simulink model "Start_Stop_ECU"  (R2023b)
settings: Solver=FixedStepDiscrete  StartTime=0.0  StopTime=24  FixedStep=0.01  RelTol=1e-3
model workspace (MATLAB code in the model file):
  | % Girişler (Inputs)
  | Start_Permission = 0;
  | Start_Button = 0;
  | Motor_RPM = 0;
  | 
  | % Çıkışlar (Outputs)
  | Mars_Motoru = 0;
  | Ignition_State = 0;
  | Target_RPM = 0;
settings Model: PacingRate=0.320000  Creator=BERKE  LastModifiedBy=BERKE
settings ConfigComp: CovEnable=on  RecordCoverage=on  CovModelRefEnable=on

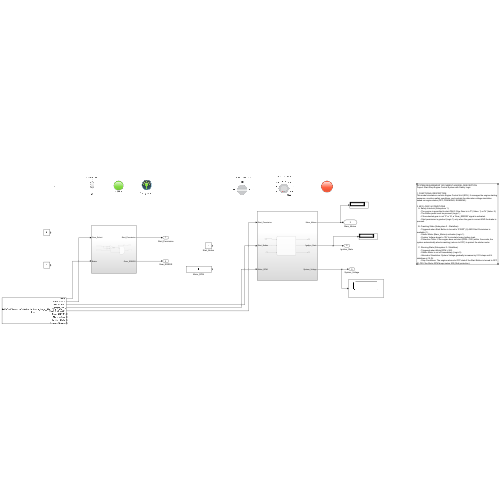
[thumbnail: Simulink's stored preview of the top-level diagram]
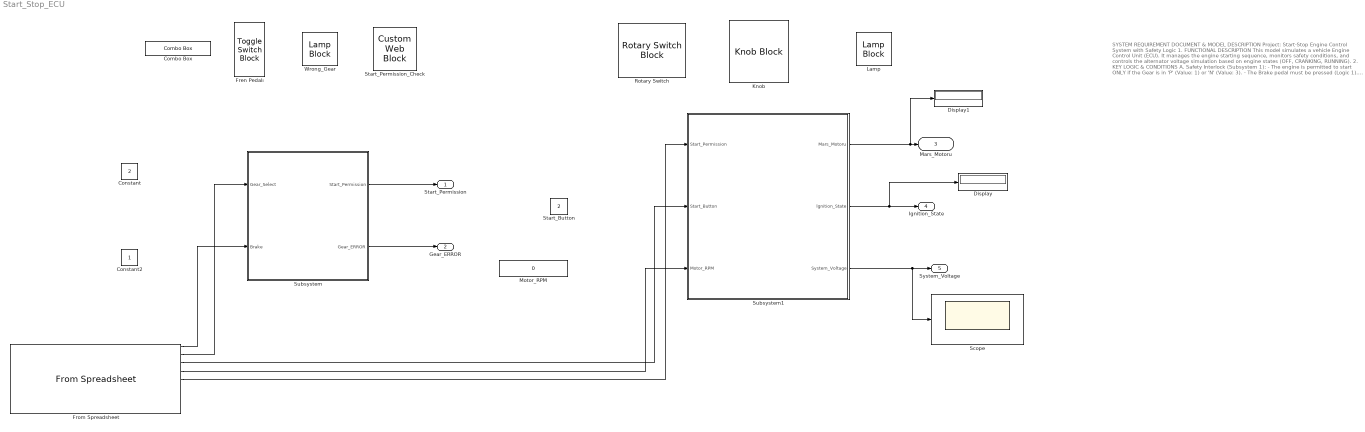
== system Start_Stop_ECU ==
  note: SYSTEM REQUIREMENT DOCUMENT & MODEL DESCRIPTION
      | Project: Start-Stop Engine Control System with Safety Logic
      |
      | 1. FUNCTIONAL DESCRIPTION
      | This model simulates a vehicle Engine Control Unit (ECU). It manages the engine starting sequence, monitors safety conditions, and controls the alternator voltage simulation based on engine states (OFF, CRANKING, RUNNING).
      |
      | 2. KEY LOGIC & CONDITIONS
      |    A. Safety Interlock (Subsystem 1):
      |       - The engine is permitted to start ONLY if the Gear is in 'P' (Value: 1) or 'N' (Value: 3).
      |       - The Brake pedal must be pressed (Logic 1).
      |       - If the selected gear is not 'P' or 'N', a 'Gear_ERROR' signal is activated.
      |       - Start permission is granted (Logic 1) only when the gear is correct AND the brake is pressed.
      |
      |    B. Cranking State (Subsystem 2 - Stateflow):
      |       - Triggered when Start Button is turned to 'START' (2) AND Start Permission is available (1).
      |       - Starter Motor (Mars_Motoru) activates (Logic 1).
      |       - System Voltage drops to 10V to simulate heavy battery load.
      |       - Protection Timer: If the engine does not start (RPM < 500) within 3 seconds, the system automatically aborts cranking (returns to OFF) to protect the starter motor.
      |
      |    C. Running State (Subsystem 2 - Stateflow):
      |       - Triggered when Motor RPM > 500.
      |       - Starter Motor is cut off immediately (Logic 0).
      |       - Alternator Simulation: System Voltage gradually increases by 0.5V steps until it stabilizes at 12.5V.
      |       - Stop Conditions: The engine returns to OFF state if the Start Button is turned to OFF (0) OR if the Motor RPM drops below 500 (Stall protection).
  Combo Box : ComboBox  LabelPosition=Hide  SelectedLabel=R
      settings: Values={{'P', 'R', 'N', 'D'}, [1 2 3 4]}
  Constant : Constant  Value=2
  Constant2 : Constant
  Display : Display
  Display1 : Display
  Fren Pedalı : ToggleSwitchBlock
      settings: Values={{'Off', 'On'}, [0 1]}
  From Spreadsheet : FromSpreadsheet  FileName=C:\Users\BERKE\OneDrive\Masaüstü\simulink\Berke_Girgin_290206067_HW2_Coverage.xlsx
  Knob : KnobBlock  ScaleMax=5000
  Lamp : LampBlock  LabelPosition=Hide
  "Motor_RPM " : Constant  Value=0
  Rotary Switch : RotarySwitchBlock
      settings: Values={{'Off', 'IGN', 'START'}, [0 1 2]}
  Scope : Scope
  Start_Button : Constant  Value=2  SampleTime=-1
  Start_Permission_Check : CustomWebBlock  LabelPosition=Bottom  ShowInitialText=on  Configuration="{\"components\":[{\"name\":\"BackgroundImageComponent\",\"settings\":{\"image\":{\"size\":[150,150],\"src\":\"data:image\\/svg+xml;base64,PHN2ZyB4bWxucz0iaHR0cDovL3d3dy53My5vcmcvMjAwMC9zdmciIHhtbG5zOnhsaW5rPSJodHRwOi8vd3d3LnczLm9yZy8xOTk5L3hsaW5rIiB2aWV3Qm94PSIwIDAgNTAwIDUwMCI+PGRlZnM+PHN0eWxlPi5he2ZpbGw6dXJsKCNhKTt9LmJ7ZmlsbDp1cmwoI2IpO30uY3tmaWxsOnVybCgjYyk7fTwvc3R5bGU+PHJhZGlhbEdyYWRpZW50IGlkPSJhIiBjeD0iMjgzLjg0IiBjeT0iLTQ2Ni4zNyIgcj0iMzc1Ljc1IiBncmFkaWVudFRyYW5zZm9ybT0ibWF0cml4KDEuMzksIDAsIDAsIC0xLjM5LCAtMTUzLjU2LCAtNjQ0LjA4KSIg ...(+2088 chars)\",\"srcOrientation\":\"Right\"},\"position\":[0,0,1,1],\"scaleMode\":\"0\"}},{\"name\":\"LampStateComponent\",\"settings\":{\"position\":[0,0,1,1],\"states\":[{\"icon\":{\"customSrc\":\"data:image\\/svg+xml;base64,PHN2ZyBpZD0iTGF5ZXJfMSIgZGF0YS1uYW1lPSJMYXllciAxIiB4bWxucz0iaHR0cDovL3d3dy53My5vcmcvMjAwMC9zdmciIHZpZXdCb3g9IjAgMCA0MTEgNDU4Ij48ZGVmcz48c3R5bGU+LmNscy0xe2ZpbGw6I2ZkZjhjMTt9LmNscy0ye2ZpbGw6I2ZlZTEwMDt9LmNscy0ze2ZpbGw6IzIzMWYyMDt9LmNscy00e2ZpbGw6I2EwOWY5Zjt9LmNscy00LC5jbHMtNSwuY2xzLTZ7c3Ryb2tlOiMyMzFmMjA7c3Ryb2tlLW1pdGVybGltaXQ6MTA7fS5jbHMtNXtmaWxsOiNmZmY7fS5jbHMtNntmaWxsOm5vbmU7fTwvc3R5bGU+PC9kZWZz ...(+5168 chars)\",\"id\":-1,\"srcOrientation\":\"Right\",\"type\":\"custom\"},\"iconScale\":0.8,\"metadata\":{},\"overlayType\":\"intersect\",\"shape\":{\"color\":[0.725,0,0],\"opacity\":1,\"position\":[0.1,0.1,0.8,0.8],\"type\":\"ellipse\"},\"value\":[]},{\"icon\":{\"customSrc\":\"data:image\\/svg+xml;base64,PHN2ZyBpZD0iTGF5ZXJfMSIgZGF0YS1uYW1lPSJMYXllciAxIiB4bWxucz0iaHR0cDovL3d3dy53My5vcmcvMjAwMC9zdmciIHZpZXdCb3g9IjAgMCA0MTEgNDU4Ij48ZGVmcz48c3R5bGU+LmNscy0xe2ZpbGw6I2ZkZjhjMTt9LmNscy0ye2ZpbGw6I2ZlZTEwMDt9LmNscy0ze2ZpbGw6IzIzMWYyMDt9LmNscy00e2ZpbGw6I2EwOWY5Zjt9LmNscy00LC5jbHMtNSwuY2xzLTZ7c3Ryb2tlOiMyMzFmMjA7c3Ryb2tlLW1pdGVybGltaXQ6MTA7fS5jbHMtNXtmaWxsOiNmZmY7fS5jbHMtNntmaWxsOm5vbmU7fTwvc3R5bGU+PC9kZWZz ...(+5168 chars)\",\"id\":-1,\"srcOrientation\":\"Right\",\"type\":\"custom\"},\"iconScale\":0.8,\"metadata\":{\"useDefaults\":{\"customIcon\":true,\"icon\":true,\"overlayType\":true,\"shape\":true,\"sizeAndPosition\":true}},\"overlayType\":\"intersect\",\"shape\":{\"color\":[0.6352941176470588,0.0784313725490196,0.1843137254901961],\"opacity\":1,\"position\":[0.1,0.1,0.8,0.8],\"type\":\"ellipse\"},\"value\":\"0\"},{\"icon\":{\"customSrc\":\"data:image\\/svg+xml;base64,PHN2ZyBpZD0iTGF5ZXJfMSIgZGF0YS1uYW1lPSJMYXllciAxIiB4bWxucz0iaHR0cDovL3d3dy53My5vcmcvMjAwMC9zdmciIHZpZXdCb3g9IjAgMCA0MTEgNDU4Ij48ZGVmcz48c3R5bGU+LmNscy0xe2ZpbGw6I2ZkZjhjMTt9LmNscy0ye2ZpbGw6I2ZlZTEwMDt9LmNscy0ze2ZpbGw6IzIzMWYyMDt9LmNscy00e2ZpbGw6I2EwOWY5Zjt9LmNscy00LC5jbHMtNSwuY2xzLTZ7c3Ryb2tlOiMyMzFmMjA7c3Ryb2tlLW1pdGVybGltaXQ6MTA7fS5jbHMtNXtmaWxsOiNmZmY7fS5jbHMtNntmaWxsOm5vbmU7fTwvc3R5bGU+PC9kZWZz ...(+5168 chars)\",\"id\":-1,\"srcOrientation\":\"Right\",\"type\":\"custom\"},\"iconScale\":0.8,\"metadata\":{\"useDefaults\":{\"customIcon\":true,\"icon\":true,\"overlayType\":true,\"shape\":true,\"sizeAndPosition\":true}},\"overlayType\":\"intersect\",\"shape\":{\"color\":[0.39215686274509803,0.8313725490196079,0.07450980392156863],\"opacity\":1,\"position\":[0.1,0.1,0.8,0.8],\"type\":\"ellipse\"},\"value\":\"1\"}],\"valueType\":\"discrete\"}},{\"name\":\"ForegroundImageComponent\",\"settings\":{\"image\":{\"size\":[150,150],\"src\":\"data:image\\/svg+xml;base64,PHN2ZyB4bWxucz0iaHR0cDovL3d3dy53My5vcmcvMjAwMC9zdmciIHhtbG5zOnhsaW5rPSJodHRwOi8vd3d3LnczLm9yZy8xOTk5L3hsaW5rIiB2aWV3Qm94PSIwIDAgNTAwIDUwMCI+PGRlZnM+PHN0eWxlPi5he2ZpbGw6dXJsKCNhKTt9PC9zdHlsZT48bGluZWFyR3JhZGllbnQgaWQ9ImEiIHgxPSIxNzMuMDUiIHkxPSItNjI3Ljc4IiB4Mj0iMTczLjA1IiB5Mj0iLTUyMi40MyIgZ3JhZGllbnRUcmFuc2Zvcm09Im1hdHJpeCgxLjI5LCAwLCAwLCAtMS4zMywgMjcuMTMsIC02MjguMzEpIiBncmFkaWVudFVuaXRzPSJ1c2VyU3BhY2VPblVzZSI+PHN0b3Agb2Zmc2V0PSIwIiBzdG9wLWNvbG9yPSIjZmZmIiBzdG9wLW9wYWNpdHk9IjAuMjUiLz48c3RvcCBvZmZzZXQ9IjEiIHN0b3AtY29sb3I9IiNmZmYiIHN0b3Atb3BhY2l0eT0iMCIvPjwvbGluZWFyR3JhZGllbnQ+PC9kZWZzPjxwYXRoIGNsYXNzPSJhIiBkPSJNNDI5LjMsMTkwLjY2QzQwMi40NSwxMTQuNTEsMzMyLjY3LDYwLjE3LDI1MC44NSw2MC4xN2MtODMuNDMsMC0xNTQuMjgsNTYuNDItMTc5Ljk1LDEzNSwxNS4zNCwzOSw4OC4xMSw3LDE3Ny4wNyw3QzM0MCwyMDIuMDgsNDE3LjI2LDIzNi40Niw0MjkuMywxOTAuNjZaIi8+PC9zdmc+\",\"srcOrientation\":\"Right\"},\"isForeground\":1,\"position\":[0,0,1,1],\"scaleMode\":\"0\"}}],\"settings\":{\"BindingType\":\"signal\",\"aspectRatio\":1.032258064516129,\"backgroundColor\":[0,0,0],\"backgroundOffset\":0.14,\"backgroundOpacity\":1,\"blockOrientation\":\"Right\",\"fixedAspectRatio\":\"on\",\"showBackgroundColor\":false,\"value\":0,\"version\":\"R2023a\"},\"type\":\"Lamp\"}"  StateValueType=Discrete  Icon=Custom
  Subsystem : Subsystem
  Subsystem1 : Subsystem
  Wrong_Gear : LampBlock  LabelPosition=Bottom
  Start_Permission : Outport
  Gear_ERROR : Outport  Port=2
  Mars_Motoru : Outport  Port=3
  Ignition_State : Outport  Port=4
  System_Voltage : Outport  Port=5
  wires:
  Subsystem/1(Start_Permission) -> Start_Permission/1
  Subsystem/2(Gear_ERROR) -> Gear_ERROR/1
  Subsystem1/1(Mars_Motoru) -> Display1/1, Mars_Motoru/1
  Subsystem1/2(İgnition_State) -> Display/1, Ignition_State/1
  Subsystem1/3(System_Voltage) -> Scope/1, System_Voltage/1
  From Spreadsheet/2 -> Subsystem/1(Gear_Select)
  From Spreadsheet/1 -> Subsystem/2(Brake)
  From Spreadsheet/3 -> Subsystem1/2(Start_Button)
  From Spreadsheet/4 -> Subsystem1/3("Motor_RPM ")
  From Spreadsheet/5 -> Subsystem1/1(Start_Permission)

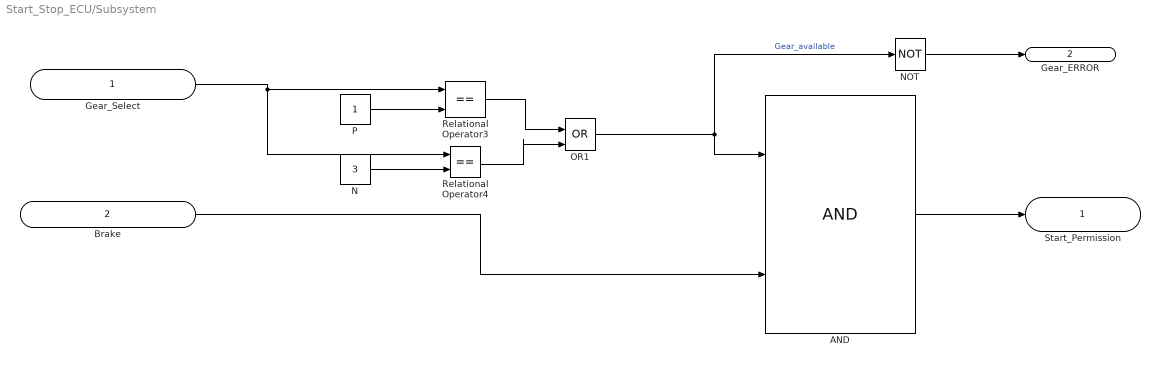
== system Start_Stop_ECU/Subsystem ==
  Gear_Select : Inport
  Brake : Inport  Port=2
  AND : Logic  IconShape=distinctive  AllPortsSameDT=off  OutDataTypeStr=boolean
  N : Constant  Value=3  SampleTime=-1
  NOT : Logic  Operator=NOT  IconShape=distinctive  AllPortsSameDT=off  OutDataTypeStr=boolean
  OR1 : Logic  Operator=OR  IconShape=distinctive  AllPortsSameDT=off  OutDataTypeStr=boolean
  P : Constant  SampleTime=-1
  Relational Operator3 : RelationalOperator  Operator===  OutDataTypeStr=boolean  RndMeth=Simplest  InputSameDT=off
  Relational Operator4 : RelationalOperator  Operator===  OutDataTypeStr=boolean  RndMeth=Simplest  InputSameDT=off
  Start_Permission : Outport
  Gear_ERROR : Outport  Port=2
  wires:
  OR1/1 -> NOT/1, AND/1  "Gear_available"
  Gear_Select/1 -> Relational Operator4/1, Relational Operator3/1
  P/1 -> Relational Operator3/2
  NOT/1 -> Gear_ERROR/1
  Relational Operator3/1 -> OR1/1
  N/1 -> Relational Operator4/2
  Relational Operator4/1 -> OR1/2
  AND/1 -> Start_Permission/1
  Brake/1 -> AND/2

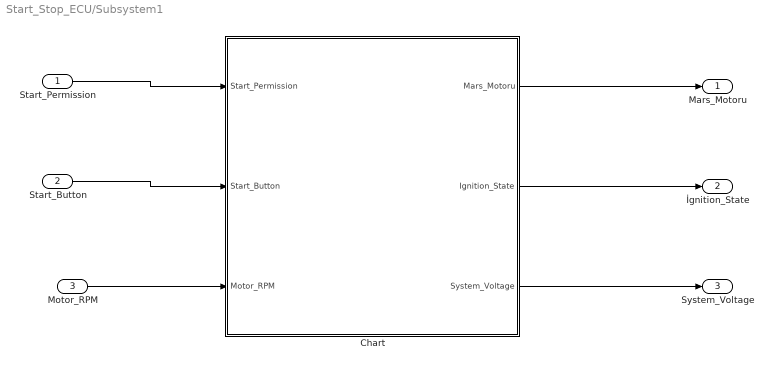
== system Start_Stop_ECU/Subsystem1 ==
  Start_Permission : Inport
  Start_Button : Inport  Port=2
  "Motor_RPM " : Inport  Port=3
  Chart : Stateflow chart  TreatAsAtomicUnit=on
  Mars_Motoru : Outport
  İgnition_State : Outport  Port=2
  System_Voltage : Outport  Port=3
  wires:
  Start_Permission/1 -> Chart/1(Start_Permission)
  Start_Button/1 -> Chart/2(Start_Button)
  Chart/1(Mars_Motoru) -> Mars_Motoru/1
  Chart/3(System_Voltage) -> System_Voltage/1
  Chart/2(Ignition_State) -> İgnition_State/1
  "Motor_RPM "/1 -> Chart/3(Motor_RPM)

== stateflow chart Start_Stop_ECU/Subsystem1/Chart ==
  settings: updateMethod=DISCRETE  sampleTime=1
  state RUNNING
    entry:
    Mars_Motoru = 0;
    Ignition_State = 1;
    System_Voltage = 10;
    during:
    if (System_Voltage < 12.5)
    System_Voltage = System_Voltage + 0.5;
    else
    System_Voltage=12.5;
    end
  state CRANKING
    entry:
    Mars_Motoru = 1;
    Ignition_State = 1;
    System_Voltage = 10;
  state OFF
    entry:
    Mars_Motoru = 0;
    Ignition_State =0;
    System_Voltage = 12;
  RUNNING -> OFF : [Start_Button == 0 || Motor_RPM < 500]
  (default) -> OFF
  CRANKING -> RUNNING [order 2] : [Motor_RPM > 500]
  OFF -> CRANKING : [Start_Button == 2 && Start_Permission == 1]
  CRANKING -> OFF [order 1] : after(3, sec)
  data: Start_Permission input; Start_Button input; Mars_Motoru output; Ignition_State output; System_Voltage output; Motor_RPM input
